simulink model "hop1a"  (R2020b)
settings: Solver=VariableStepAuto  StartTime=0.0  StopTime=1000  RelTol=1e-3
libraries: simulink x2
settings Model: EnablePacing=on  Creator=stefanopanzieri  LastModifiedBy=Stefano

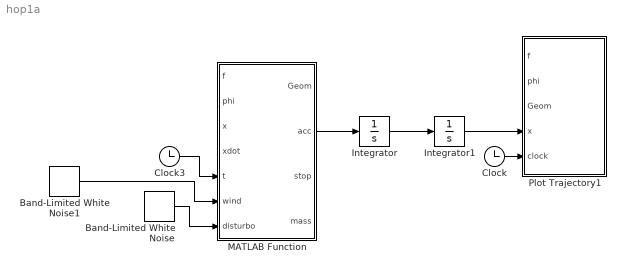
== system hop1a ==
  Band-Limited White Noise : simulink/Sources/Band-Limited White Noise  Cov=[0.000001]  Ts=0.1  seed=[23341]
  Band-Limited White Noise1 : simulink/Sources/Band-Limited White Noise  Cov=[0.000000001]  Ts=0.1  seed=[23341]
  Clock : Clock
  Clock3 : Clock
  Integrator : Integrator  InitialCondition=[0 0 0]
  Integrator1 : Integrator  InitialCondition="[0 20  0]"
  MATLAB Function : MATLAB Function  TreatAsAtomicUnit=on  SystemSampleTime=0.01
  Plot Trajectory1 : MATLAB Function  TreatAsAtomicUnit=on  SystemSampleTime=0.1
  wires:
  Integrator/1 -> Integrator1/1
  MATLAB Function/2(acc) -> Integrator/1
  Clock/1 -> Plot Trajectory1/5(clock)
  Integrator1/1 -> Plot Trajectory1/4(x)
  Clock3/1 -> MATLAB Function/5(t)
  Band-Limited White Noise1/1 -> MATLAB Function/6(wind)
  Band-Limited White Noise/1 -> MATLAB Function/7(disturbo)

== matlab function hop1a/Plot Trajectory1 ==
  settings: updateMethod=DISCRETE
  data: f input; phi input; Geom input; x input; clock input
function PlotRocket(f,phi,Geom,x,clock)

eml.extrinsic('findobj','get','set','figure','clf',...
              'hold','delete','plot','axis','grid',...
              'hggroup','quiver','drawnow');
          
persistent chain;
persistent thrust;
persistent ground;
persistent deleted_fig;

L=Geom(1);
Alt=Geom(2);
Dia=Geom(3);

% posizione del propulsore
pex=x(1)+L*sin(x(3));
pey=x(2)-L*cos(x(3));

% Vettore di propulsione
vex=f*sin(x(3)+phi)/2000;
vey=-f*cos(x(3)+phi)/2000;

          
% Gestisco la figura di output
if isempty(deleted_fig)
    deleted_fig=1;
    % La prima volta cancello la figura
    foundFig=findobj('Tag','trajScope');
    if ~isempty(foundFig)
        cla(foundFig)
        %foundFig=findobj('Tag','stroboScope');
    end      
else
    foundFig=findobj('Tag','trajScope');
end



if isempty(foundFig)
    fig=figure('Color','white');
    clf(fig);
    set(fig,'Name','Trajectory');
    set(fig,'DoubleBuffer','on','Tag','trajScope');
    set(fig,'Renderer','painters');
    hold('on');
    hax=get(fig,'CurrentAxes');
    set(hax,'DrawMode','fast','Box','off');    
    

    chain=hggroup;
    thrust=quiver(hax,pex,pey,vex,vey,'Color','green','LineWidth',2);
    ground=plot([-30 30],[0 0],'c','LineWidth',3);
    grid('on');
    
else
    
    hax=get(foundFig,'CurrentAxes');

end


if ~isempty(chain)
    delete(chain);
    delete(thrust);
end



% draw the center of mass
chain=hggroup;
h1=plot(hax,x(1),x(2),'r*','LineWidth',3);


width = Dia; % whatever
height = Alt; % whatever...
xLeft = - width/2;
xRigth = width/2;
yBottom = - L;
yTop = height;
xPoint=0;
yPoint=height*3/2;

Vertex=[xLeft yTop  1
        xPoint yPoint 1
        xRigth yTop  1
        xRigth yBottom 1
        xLeft  yBottom 1
        xLeft yTop  1];
    
Rot=[cos(-x(3))  sin(-x(3)) x(1)
     -sin(-x(3)) cos(-x(3)) x(2)
      0         0        1];
      
Vertex=(Rot*Vertex')';

h2=line(Vertex(:,1),Vertex(:,2));


%h2=rectangle('Position', [xLeft, yBottom, width, height], 'EdgeColor', 'b', 'FaceColor', 'r', 'LineWidth', 4);

set(h1,'Parent',chain);
set(h2,'Parent',chain);



% draw the thrust

thrust=quiver(hax,pex,pey,vex,vey,'Color','green','LineWidth',2);


% draw the ground
if x(2)<100
    if isempty(ground)
        ground=plot([-30 30],[0 0],'c','LineWidth',3);
    end
end



%axis([-2 42 0 102])
axis equal
drawnow;

== matlab function hop1a/MATLAB Function ==
  data: Geom output; f input; acc output; phi input; x input; xdot input; stop output; t input; wind input; disturbo input; mass output
function [Geom,acc,stop,mass] = accelerazioni(f,phi,x,xdot,t,wind,disturbo)

% y: spostamento laterale x(1)
% z:   quota x(2)
% theta: angolo razzo x(3)
% phi: angolo di controllo dell'ugello
% f: spinta del razzo

persistent mass_consumption;

Geom=[0 0 0];
stop=0;
acc=[0 0 0];
mass=0;

if t<20
    disturbo=0;
end

M=45000;  % peso in Kg 
Dia=9; % diametro 
Alt=50; % altezza 
I=1/12*M*(Dia^2+Alt^2); % inerzia in Kg*m^2
L=20;    % distanza baricentro-ugello
g=9.8;  % accelerazione di gravitÃ 
D=M*g/100; % attrito necessario a cadere al massimo a 350 Km/h
Specific_Impulse=334; % Impulso specifico
Flow_Rate=931.2; % sea level
Fmax=(Flow_Rate*Specific_Impulse)*3; % 3 raptors


acc(1)= -f*sin(x(3)+phi)/M+wind; 
acc(2)= -g + f/M*cos(x(3) + phi) - D/M*xdot(2);      
acc(3)= -L/I*sin(phi)*f+disturbo;


% Consumo della massa
if isempty(mass_consumption)
   mass_consumption=0; 
end
%mass_consumption=mass_consumption+0.01*(f/Fmax)*932.2;
mass_consumption=mass_consumption+0.01*f/(Specific_Impulse*3);

mass=M-mass_consumption;


% Stop alla simulazione
if x(2)<=L & t>10
     stop=1;
end
% 

% Sulla piattaforma di lancio non può andare indietro
if x(2)<L & acc(2)<0
     acc(2)=0;
end


Geom(1)=L;
Geom(2)=Alt;
Geom(3)=Dia;
